simulink model "reflexStiffnessLPVModel"  (Simulink 8.2)
settings: Solver=ode3  StartTime=0.0  StopTime=simulationTime  FixedStep=0.001  RelTol=1e-3
values from neighbouring files (symbols this model uses):
  simulationSamplingTime = 0.001    [simLPV_ParallelCascade.m]    (also in simulate_LPV_ParallelCascade.m)
libraries: dsppolyfun x1
settings Model: Creator=Kian  LastModifiedBy=Kian
settings DataIOCC: SignalLoggingSaveFormat=Dataset
settings OptimizationCC: ExpressionDepthLimit=128
settings DebuggingCC: FcnCallInpInsideContextMsg=EnableAllAsError  StateNameClashWarn=none
settings GRTTargetCC: CombineOutputUpdateFcns=on  GRTInterface=off

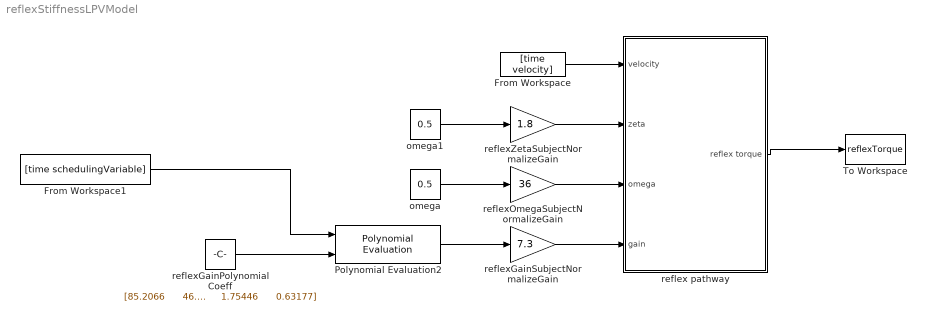
== system reflexStiffnessLPVModel ==
  From Workspace : FromWorkspace  VariableName=[time velocity]  SampleTime=simulationSamplingTime
  From Workspace1 : FromWorkspace  VariableName=[time schedulingVariable]  SampleTime=simulationSamplingTime
  Polynomial Evaluation2 : dsppolyfun/Polynomial Evaluation  useConstCoeffs=off  constCoeffs=[5 4 3 2 1]
  To Workspace : ToWorkspace  VariableName=reflexTorque  SampleTime=simulationSamplingTime
  omega : Constant  Value=0.5
  omega1 : Constant  Value=0.5
  reflex pathway : Subsystem
  reflexGainPolynomialCoeff : Constant  Value="[85.2066      46.2746     -10.9566     -5.30716      1.75446      0.63177]"
  reflexGainSubjectNormalizeGain : Gain  Gain=7.3
  reflexOmegaSubjectNormalizeGain : Gain  Gain=36
  reflexZetaSubjectNormalizeGain : Gain  Gain=1.8
  wires:
  From Workspace/1 -> reflex pathway/1(velocity)
  reflex pathway/1(reflex torque) -> To Workspace/1
  From Workspace1/1 -> Polynomial Evaluation2/1
  omega1/1 -> reflexZetaSubjectNormalizeGain/1
  omega/1 -> reflexOmegaSubjectNormalizeGain/1
  reflexZetaSubjectNormalizeGain/1 -> reflex pathway/2(zeta)
  reflexOmegaSubjectNormalizeGain/1 -> reflex pathway/3(omega)
  reflexGainSubjectNormalizeGain/1 -> reflex pathway/4(gain)
  reflexGainPolynomialCoeff/1 -> Polynomial Evaluation2/2
  Polynomial Evaluation2/1 -> reflexGainSubjectNormalizeGain/1

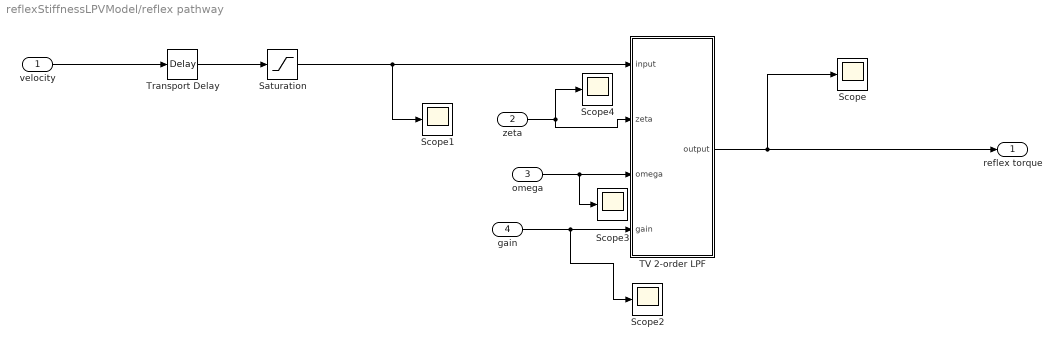
== system reflexStiffnessLPVModel/reflex pathway ==
  velocity : Inport
  zeta : Inport  Port=2
  omega : Inport  Port=3
  gain : Inport  Port=4
  Saturation : Saturate  UpperLimit=Inf  LowerLimit=0
  Scope{,1..4} (5 alike) : Scope
      Scope settings: YMin=-3500  YMax=1250
      Scope2 settings: SaveName=ScopeData2
      Scope3 settings: SaveName=ScopeData3
      Scope4 settings: YMin=0.9  YMax=0.9  SaveName=ScopeData4
  TV 2-order LPF : Subsystem
  Transport Delay : TransportDelay  DelayTime=0.04
  reflex torque : Outport
  wires:
  TV 2-order LPF/1(output) -> reflex torque/1, Scope/1
  velocity/1 -> Transport Delay/1
  Saturation/1 -> Scope1/1, TV 2-order LPF/1(input)
  Transport Delay/1 -> Saturation/1
  zeta/1 -> TV 2-order LPF/2(zeta), Scope4/1
  gain/1 -> Scope2/1, TV 2-order LPF/4(gain)
  omega/1 -> Scope3/1, TV 2-order LPF/3(omega)

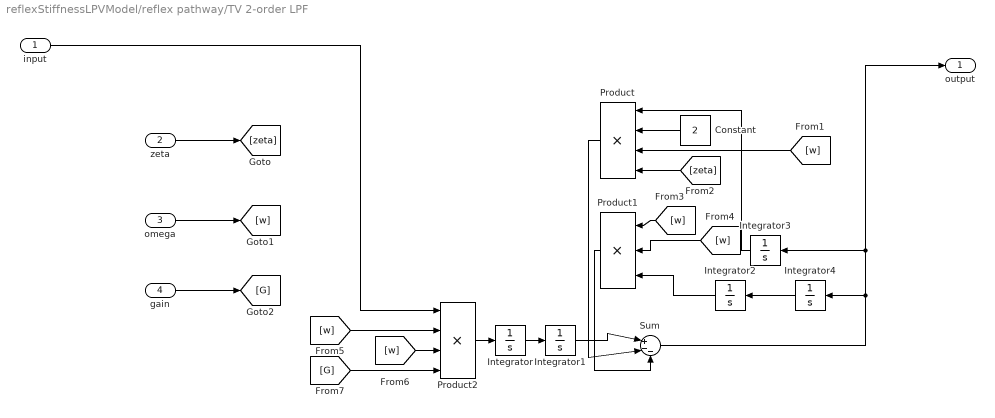
== system reflexStiffnessLPVModel/reflex pathway/TV 2-order LPF ==
  input : Inport
  zeta : Inport  Port=2
  omega : Inport  Port=3
  gain : Inport  Port=4
  Constant : Constant  Value=2
  Integrator{,1..4} (5 alike) : Integrator
  Product : Product  Inputs=4
  Product1 : Product  Inputs=3
  Product2 : Product  Inputs=4
  Sum : Sum  Inputs=|+--
  output : Outport
  wires:
  Integrator1/1 -> Sum/1
  Integrator/1 -> Integrator1/1
  Product2/1 -> Integrator/1
  Integrator3/1 -> Product/1
  Integrator2/1 -> Product1/3
  Sum/1 -> Integrator4/1, output/1, Integrator3/1
  Integrator4/1 -> Integrator2/1
  input/1 -> Product2/1
  gain/1 -> [G]
  Product1/1 -> Sum/3
  [w] -> Product2/3
  [w] -> Product2/2
  Constant/1 -> Product/2
  [w] -> Product1/1
  Product/1 -> Sum/2
  [w] -> Product/3
  zeta/1 -> [zeta]
  [zeta] -> Product/4
  [w] -> Product1/2
  [G] -> Product2/4
  omega/1 -> [w]
